simulink library "csu_cml_command_latch_lib"  (R2015b)
settings: Solver=ode45  StartTime=0.0  StopTime=10.0  RelTol=1e-3
values from neighbouring files (symbols this model uses):
  cml_mode_ids = zeros(size(cml_valid_modes))    [csu_cml_command_latch_init.m]
  cml_valid_mode_transitions = zeros(n, 'uint8')    [csu_cml_command_latch_init.m]
  csc_cmp_dt = fsw_dt    [csc_cmp_command_mode_process_init.m]
undefined symbols (not defined in the file or in its folder): cml_cmd_indices, cml_initial_value, cmp_msgid
libraries: simulink x8, util_event_lib x5, util_info_lib x1
settings Model: Creator=mstewart  LastModifiedBy=Mark Agbayani
settings DataIOCC: SaveFormat=Array
settings DebuggingCC: UnderspecifiedInitializationDetection=Classic  MergeDetectMultiDrivingBlocksExec=none  SolverPrmCheckMsg=warning  StateNameClashWarn=warning
settings HardwareCC: ProdBitPerPointer=32  ProdLargestAtomicFloat=None  ProdIntDivRoundTo=Undefined  ProdEndianess=Unspecified  ProdWordSize=32  ProdHWDeviceType=32-bit Generic
settings GRTTargetCC: GeneratePreprocessorConditionals=Disable all
settings ConfigComp: CovModelRefEnable=Off  CovSFcnEnable=off

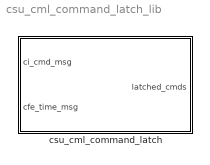
== system csu_cml_command_latch_lib ==
  csu_cml_command_latch : Subsystem

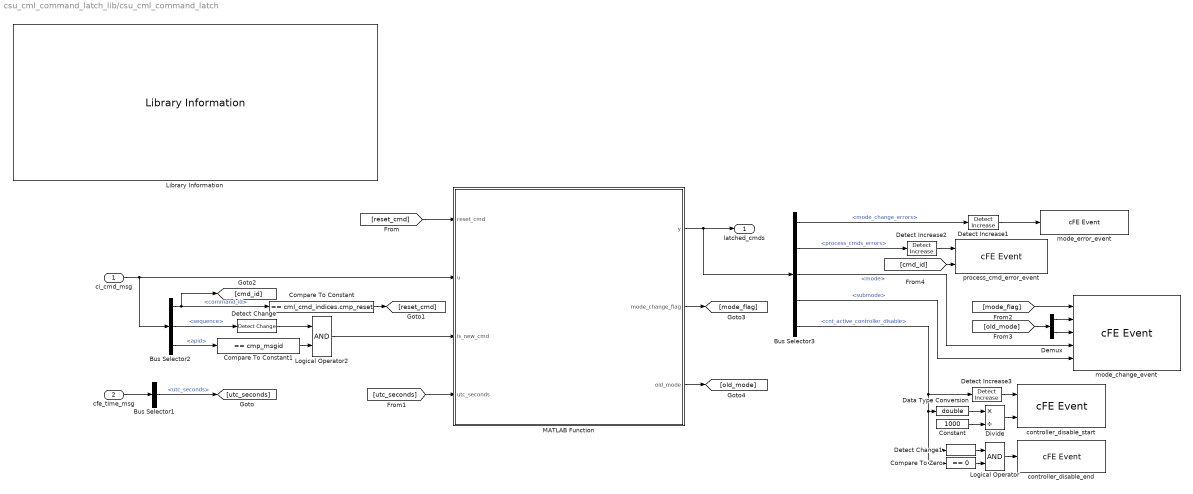
== system csu_cml_command_latch_lib/csu_cml_command_latch ==
  ci_cmd_msg : Inport  OutDataTypeStr=Bus: ci_cmd_msg
  cfe_time_msg : Inport  Port=2  OutDataTypeStr=Bus: cfe_time_msg
  Bus Selector1 : BusSelector  OutputSignals=utc_seconds
  Bus Selector2 : BusSelector  OutputSignals=command_id,sequence,apid
  Bus Selector3 : BusSelector  OutputSignals=mode_change_errors,process_cmds_errors,mode,submode,cnt_active_controller_disable
  Compare To Constant : simulink/Logic and Bit Operations/Compare To Constant  relop===  const=cml_cmd_indices.cmp_reset  OutDataTypeStr=boolean
  Compare To Constant1 : simulink/Logic and Bit Operations/Compare To Constant  relop===  const=cmp_msgid  OutDataTypeStr=boolean
  Compare To Zero : simulink/Logic and Bit Operations/Compare To Zero  relop===  OutDataTypeStr=boolean
  Constant : Constant  Value=1000  OutDataTypeStr=double
  Data Type Conversion : DataTypeConversion  OutDataTypeStr=double
  Demux : Demux  Outputs=2
  Detect Change : simulink/Logic and Bit Operations/Detect Change  vinit=0  InputProcessing=Inherited  OutDataTypeStr=boolean
  Detect Change1 : simulink/Logic and Bit Operations/Detect Change  vinit=0  InputProcessing=Inherited  OutDataTypeStr=boolean
  Detect Increase1 : simulink/Logic and Bit Operations/Detect Increase  vinit=0.0  InputProcessing=Inherited  OutDataTypeStr=boolean
  Detect Increase2 : simulink/Logic and Bit Operations/Detect Increase  vinit=0.0  InputProcessing=Inherited  OutDataTypeStr=boolean
  Detect Increase3 : simulink/Logic and Bit Operations/Detect Increase  vinit=0.0  InputProcessing=Inherited  OutDataTypeStr=boolean
  Divide : Product  Inputs=*/
  Library Information : util_info_lib/Library Information  owner='NONE'
  Logical Operator : Logic  AllPortsSameDT=off  OutDataTypeStr=boolean
  Logical Operator2 : Logic  AllPortsSameDT=off  OutDataTypeStr=boolean
  MATLAB Function : MATLAB Function  TreatAsAtomicUnit=on
  controller_disable_end : util_event_lib/cFE Event  event_message='Active Control Re-enabled'  event_id=24  event_severity=INFORMATION  event_filtered=off  event_mask=1  event_use_enums=off  event_enum_types={}
  controller_disable_start : util_event_lib/cFE Event  event_message='Active Control Disabled for %f seconds'  event_id=23  event_severity=INFORMATION  event_filtered=off  event_mask=1  event_use_enums=off  event_enum_types={}
  mode_change_event : util_event_lib/cFE Event  event_message='Mode changed from %s:%s to %s:%s'  event_id=20  event_severity=INFORMATION  event_filtered=off  event_mask=1  event_use_enums=on  event_enum_types={'enum_mode', 'enum_submode', 'enum_mode', 'enum_submode'}
  mode_error_event : util_event_lib/cFE Event  event_message='Invalid mode change requested'  event_id=22  event_severity=ERROR  event_filtered=off  event_mask=1  event_use_enums=off  event_enum_types={}
  process_cmd_error_event : util_event_lib/cFE Event  event_message='Error processing command with command code %u'  event_id=21  event_severity=ERROR  event_filtered=off  event_mask=1  event_use_enums=off  event_enum_types={}
  latched_cmds : Outport  OutDataTypeStr=Bus: cmp_bus_msg
  wires:
  Constant/1 -> Divide/2
  Data Type Conversion/1 -> Divide/1
  Divide/1 -> controller_disable_start/2
  Logical Operator/1 -> controller_disable_end/1
  Compare To Zero/1 -> Logical Operator/2
  Detect Change1/1 -> Logical Operator/1
  Bus Selector3/5 -> Detect Increase3/1, Compare To Zero/1, Detect Change1/1, Data Type Conversion/1  "<cnt_active_controller_disable>"
  Detect Increase3/1 -> controller_disable_start/1
  [old_mode] -> Demux/1
  [mode_flag] -> mode_change_event/1
  MATLAB Function/2(mode_change_flag) -> [mode_flag]
  Bus Selector3/4 -> mode_change_event/5  "<submode>"
  Bus Selector3/3 -> mode_change_event/4  "<mode>"
  Demux/2 -> mode_change_event/3
  Demux/1 -> mode_change_event/2
  ci_cmd_msg/1 -> MATLAB Function/2(u), Bus Selector2/1
  MATLAB Function/1(y) -> Bus Selector3/1, latched_cmds/1
  cfe_time_msg/1 -> Bus Selector1/1
  Bus Selector1/1 -> [utc_seconds]  "<utc_seconds>"
  Bus Selector2/1 -> [cmd_id], Compare To Constant/1  "<command_id>"
  Compare To Constant/1 -> [reset_cmd]
  Bus Selector2/2 -> Detect Change/1  "<sequence>"
  [reset_cmd] -> MATLAB Function/1(reset_cmd)
  [utc_seconds] -> MATLAB Function/4(utc_seconds)
  Logical Operator2/1 -> MATLAB Function/3(is_new_cmd)
  Bus Selector3/2 -> Detect Increase2/1  "<process_cmds_errors>"
  [cmd_id] -> process_cmd_error_event/2
  Detect Increase2/1 -> process_cmd_error_event/1
  Bus Selector3/1 -> Detect Increase1/1  "<mode_change_errors>"
  Detect Increase1/1 -> mode_error_event/1
  Bus Selector2/3 -> Compare To Constant1/1  "<apid>"
  Detect Change/1 -> Logical Operator2/1
  Compare To Constant1/1 -> Logical Operator2/2
  MATLAB Function/3(old_mode) -> [old_mode]

== matlab function csu_cml_command_latch_lib/csu_cml_command_latch/MATLAB Function ==
  data: csc_cmp_dt parameter; reset_cmd input boolean; u input Bus: ci_cmd_msg; y output Bus: cmp_bus_msg; is_new_cmd input boolean; utc_seconds input uint32; mode_change_flag output uint8; cml_valid_mode_transitions parameter; cml_mode_ids parameter uint8; cml_cmd_indices parameter; old_mode output uint8; cml_initial_value parameter
function [y, mode_change_flag, old_mode] = decode_and_latch(csc_cmp_dt, reset_cmd, u, is_new_cmd, utc_seconds, cml_valid_mode_transitions, cml_mode_ids, cml_cmd_indices, cml_initial_value)
%#codegen

persistent latched_values;
persistent internal_counters;

if isempty(latched_values)
    % load in inital values for all command signals
    latched_values = cml_initial_value;
end

if isempty(internal_counters)
    internal_counters.start_burn_count = uint8(0);
    internal_counters.old_mode = uint8( 1 );
    internal_counters.old_submode = uint8( 1 );
    internal_counters.controller_disable_counter = uint32( 0 );
    internal_counters.manual_thruster_duration_counter = uint32( zeros(26,1) );
    internal_counters.manual_thruster_arm_duration_counter = uint32( zeros(4,1) );
    internal_counters.act_reset = uint8(0);
end


if internal_counters.start_burn_count > 0
    internal_counters.start_burn_count = internal_counters.start_burn_count - 1;
    if internal_counters.start_burn_count == 0
        latched_values.start_burn = uint8(0);
    end
end

if internal_counters.act_reset > 0
    internal_counters.act_reset = internal_counters.act_reset - 1;
    if internal_counters.act_reset == 0
        latched_values.act_reset_accumulated_ontime = uint8(0);
    end
end

if internal_counters.controller_disable_counter > 0
    internal_counters.controller_disable_counter = internal_counters.controller_disable_counter - 100;
    if internal_counters.controller_disable_counter == 0
        latched_values.cnt_active_controller_disable = uint32(0);
    else
        latched_values.cnt_active_controller_disable = internal_counters.controller_disable_counter;
    end
end

if any(internal_counters.manual_thruster_duration_counter > 0)
    internal_counters.manual_thruster_duration_counter = max(internal_counters.manual_thruster_duration_counter - 100, uint32(zeros(26,1)));
    if all( internal_counters.manual_thruster_duration_counter == 0 )
        latched_values.act_manual_thruster_firing = uint32(zeros(26,1));
        internal_counters.manual_thruster_duration_counter = uint32(zeros(26,1));
    else
        latched_values.act_manual_thruster_firing = internal_counters.manual_thruster_duration_counter;
    end
end

if any(internal_counters.manual_thruster_arm_duration_counter > 0)
    internal_counters.manual_thruster_arm_duration_counter = max(internal_counters.manual_thruster_arm_duration_counter - 100, uint32(zeros(4,1)));
    if all( internal_counters.manual_thruster_arm_duration_counter == 0 )
        latched_values.act_arm_thruster_set_durations = uint32(zeros(4,1));
        internal_counters.manual_thruster_arm_duration_counter = uint32(zeros(4,1));
    else
        latched_values.act_arm_thruster_set_durations = internal_counters.manual_thruster_arm_duration_counter;
    end
end

old_mode = [ latched_values.mode latched_values.submode];
mode_change_flag = uint8( 0 );

if is_new_cmd
    
    latched_values.command_id = uint8(u.command_id);

    %%% Handle mode commands
    if (u.command_id == cml_cmd_indices.cmp_set_mode)

        new_mode = typecast(u.params(1),'uint8');   % decode requested "new mode"
        new_submode = typecast(u.params(2),'uint8');   % decode requested "new submode"
        
        if new_mode >= 1 && new_mode <= 9
            new_mode_id = cml_mode_ids(new_mode, new_submode);
            
            if new_mode_id ~= 0
                old_mode_id = cml_mode_ids(old_mode(1), old_mode(2));
                valid_mode_change = cml_valid_mode_transitions(old_mode_id, new_mode_id);
            else
                valid_mode_change = uint8(0);
            end
        else
            valid_mode_change = uint8(0);
        end

        if valid_mode_change                        % change modes

            latched_values.mode = new_mode;
            latched_values.submode = new_submode;
            
            if new_mode ~= internal_counters.old_mode || new_submode ~= internal_counters.old_submode
                mode_change_flag = uint8( 1 );
            end
            
            internal_counters.old_mode = new_mode;
            internal_counters.old_submode = new_submode;

            latched_values.mode_change_counter = latched_values.mode_change_counter + 1;

            if latched_values.cnt_active_controller_disable > 0     % If necessary, disable active_controller_disable
               latched_values.cnt_active_controller_disable = uint32(0);
               internal_counters.controller_disable_counter = uint32(0);
            end
            
            % If necessary, zero out current manual thruster commands
            if any(internal_counters.manual_thruster_duration_counter > 0)  || any(internal_counters.manual_thruster_arm_duration_counter > 0)
                latched_values.act_arm_thruster_set_durations = uint32(zeros(4,1));
                internal_counters.manual_thruster_arm_duration_counter = uint32(zeros(4,1));
                
                latched_values.act_manual_thruster_firing = uint32(zeros(26,1));
                internal_counters.manual_thruster_duration_counter = uint32(zeros(26,1));
            end

        else                                          % Invalid mode transition commanded, increment mode change errors counter

            latched_values.mode_change_errors = latched_values.mode_change_errors + 1;

        end                                           % Increment commands processed counter

        latched_values.process_cmds_counter = latched_values.process_cmds_counter + 1;

    elseif (u.command_id == cml_cmd_indices.cmp_disable_active_controller)
        latched_values.cnt_active_controller_disable = typecast(u.params(1:4),'uint32');
        internal_counters.controller_disable_counter = latched_values.cnt_active_controller_disable;
        
        % If necessary, zero out current manual thruster commands
        if any(internal_counters.manual_thruster_duration_counter > 0)  || any(internal_counters.manual_thruster_arm_duration_counter > 0)      
            latched_values.act_arm_thruster_set_durations = uint32(zeros(4,1));
            internal_counters.manual_thruster_arm_duration_counter = uint32(zeros(4,1));
            
            latched_values.act_manual_thruster_firing = uint32(zeros(26,1));
            internal_counters.manual_thruster_duration_counter = uint32(zeros(26,1));
        end
        
    elseif (u.command_id == cml_cmd_indices.cmp_reset_ctrs)
        latched_values.process_cmds_counter = uint16(0);
        latched_values.process_cmds_errors = uint16(0);
        latched_values.mode_change_counter = uint16(0);
        latched_values.mode_change_errors = uint16(0);
        
    elseif (u.command_id == cml_cmd_indices.gdn_hover_enable)
        latched_values.hover_enable = uint8(1);
        latched_values.process_cmds_counter = latched_values.process_cmds_counter + 1;
        
    elseif (u.command_id == cml_cmd_indices.gdn_hover_disable)
        latched_values.hover_enable = uint8(0);
        latched_values.process_cmds_counter = latched_values.process_cmds_counter + 1;
        
    elseif (u.command_id == cml_cmd_indices.gdn_takeoff_enable)
        latched_values.takeoff_enable = uint8(1);
        latched_values.process_cmds_counter = latched_values.process_cmds_counter + 1;
        
    elseif (u.command_id == cml_cmd_indices.gdn_takeoff_disable)
        latched_values.takeoff_enable = uint8(0);
        latched_values.process_cmds_counter = latched_values.process_cmds_counter + 1;
        
    elseif (u.command_id == cml_cmd_indices.gdn_set_burn_parameters)
        burn_type = typecast(u.params(1),'uint8');
        delta_v = typecast(u.params(2:9),'double');
        burn_dur = typecast(u.params(10:13),'single');
        
        if burn_type == 0 || burn_type == 1 || burn_type == 2 || burn_type == 3
            latched_values.burn_type_cmd = burn_type;
            latched_values.thruster_dv_cmd = delta_v;
            latched_values.thruster_dur_cmd = burn_dur;
        else
            latched_values.process_cmds_errors = latched_values.process_cmds_errors + 1;
        end
        
        latched_values.process_cmds_counter = latched_values.process_cmds_counter + 1;
        
    elseif (u.command_id == cml_cmd_indices.gdn_start_burn)
        
        if 1
            latched_values.start_burn = uint8(1);
            internal_counters.start_burn_count = uint8(1/csc_cmp_dt);
        else
            latched_values.process_cmds_errors = latched_values.process_cmds_errors + 1;
        end
        
        latched_values.process_cmds_counter = latched_values.process_cmds_counter + 1;
        
	elseif (u.command_id == cml_cmd_indices.gdn_set_inertial_primary_pointing_cmd)
        v_x = typecast(u.params(1:8),'double');
        v_y = typecast(u.params(9:16),'double');
        v_z = typecast(u.params(17:24),'double');
        
        if 1 % TODO: real error checking
            latched_values.inertial_primary_pointing_cmd = [v_x; v_y; v_z];
        else
            latched_values.process_cmds_errors = latched_values.process_cmds_errors + 1;
        end
        
        latched_values.process_cmds_counter = latched_values.process_cmds_counter + 1;
        
	elseif (u.command_id == cml_cmd_indices.gdn_set_inertial_secondary_pointing_cmd)
        v_x = typecast(u.params(1:8),'double');
        v_y = typecast(u.params(9:16),'double');
        v_z = typecast(u.params(17:24),'double');
        
        if 1 % TODO: real error checking
            latched_values.inertial_secondary_pointing_cmd = [v_x; v_y; v_z];
        else
            latched_values.process_cmds_errors = latched_values.process_cmds_errors + 1;
        end
        
        latched_values.process_cmds_counter = latched_values.process_cmds_counter + 1;
        
	elseif (u.command_id == cml_cmd_indices.gdn_set_body_secondary_pointing_vector)
        v_x = typecast(u.params(1:8),'double');
        v_y = typecast(u.params(9:16),'double');
        v_z = typecast(u.params(17:24),'double');
        
        if 1 % TODO: real error checking
            latched_values.body_secondary_pointing_vector = [v_x; v_y; v_z];
        else
            latched_values.process_cmds_errors = latched_values.process_cmds_errors + 1;
        end
        
        latched_values.process_cmds_counter = latched_values.process_cmds_counter + 1;
        
	elseif (u.command_id == cml_cmd_indices.gdn_set_body_primary_pointing_vector)
        v_x = typecast(u.params(1:8),'double');
        v_y = typecast(u.params(9:16),'double');
        v_z = typecast(u.params(17:24),'double');
        
        if 1 % TODO: real error checking
            latched_values.body_primary_pointing_vector = [v_x; v_y; v_z];
        else
            latched_values.process_cmds_errors = latched_values.process_cmds_errors + 1;
        end
        
        latched_values.process_cmds_counter = latched_values.process_cmds_counter + 1;
        
	elseif (u.command_id == cml_cmd_indices.gdn_set_peg_position_target)
        frame = typecast(u.params(1),'uint8');
        v_x = typecast(u.params(2:9),'double');
        v_y = typecast(u.params(10:17),'double');
        v_z = typecast(u.params(18:25),'double');
        
        if frame == 1 || frame == 3
            latched_values.peg_target_ref_frame = frame;
            latched_values.peg_position_target = [v_x; v_y; v_z];
        else
            latched_values.process_cmds_errors = latched_values.process_cmds_errors + 1;
        end
        
        latched_values.process_cmds_counter = latched_values.process_cmds_counter + 1;
                
	elseif (u.command_id == cml_cmd_indices.gdn_set_peg_velocity_target)
        frame = typecast(u.params(1),'uint8');
        v_x = typecast(u.params(2:9),'double');
        v_y = typecast(u.params(10:17),'double');
        v_z = typecast(u.params(18:25),'double');
        
        if frame == 1 || frame == 4
            latched_values.peg_target_ref_frame = frame;
            latched_values.peg_velocity_target = [v_x; v_y; v_z];
        else
            latched_values.process_cmds_errors = latched_values.process_cmds_errors + 1;
        end
        
        latched_values.process_cmds_counter = latched_values.process_cmds_counter + 1;
                
	elseif (u.command_id == cml_cmd_indices.gdn_set_vnc_primary_pointing_cmd)
        el = typecast(u.params(1:8),'double');
        az = typecast(u.params(9:16),'double');
        
        if 1 % TODO: real error checking
            latched_values.vnc_primary_pointing_cmd = [el; az];
        else
            latched_values.process_cmds_errors = latched_values.process_cmds_errors + 1;
        end
        
        latched_values.process_cmds_counter = latched_values.process_cmds_counter + 1;
        
    elseif (u.command_id == cml_cmd_indices.est_set_reference_frame)
        frame = typecast(u.params(1),'uint8');
        
        if 1 % TODO: real error checking
            latched_values.est_ref_frame = frame;
        else
            latched_values.process_cmds_errors = latched_values.process_cmds_errors + 1;
        end
        
        latched_values.process_cmds_counter = latched_values.process_cmds_counter + 1;
        
    elseif (u.command_id == cml_cmd_indices.cnt_select_thruster_set)
        thrusters = typecast(u.params(1),'uint8');
        
        if 1 % TODO: real error checking
            latched_values.acs_thruster_set = thrusters;
        else
            latched_values.process_cmds_errors = latched_values.process_cmds_errors + 1;
        end
        
        latched_values.process_cmds_counter = latched_values.process_cmds_counter + 1;
        
    
    elseif (u.command_id == cml_cmd_indices.act_fire_single_thruster)
        thruster_id = typecast(u.params(1),'uint8');
        duration = typecast(u.params(2:5),'uint32');
        
        if thruster_id > 0 && thruster_id <= 26 % TODO: real error checking

            latched_values.act_manual_thruster_firing(thruster_id) = uint32( duration );
                        
            internal_counters.manual_thruster_duration_counter = latched_values.act_manual_thruster_firing;
        else
            latched_values.act_manual_thruster_firing = uint32( zeros(26,1) );
        end
        
        latched_values.process_cmds_counter = latched_values.process_cmds_counter + 1;
        
    elseif (u.command_id == cml_cmd_indices.act_enable_thruster_set)

        thruster_set_id = typecast(u.params(1),'uint8');
        duration = typecast(u.params(2:5),'uint32');
        
        if thruster_set_id > 0 && thruster_set_id <= 4 % TODO: real error checking
            latched_values.act_arm_thruster_set_durations(thruster_set_id) = uint32( duration );
                        
            internal_counters.manual_thruster_arm_duration_counter = latched_values.act_arm_thruster_set_durations;
        else
            latched_values.act_arm_thruster_set_durations = uint32( zeros(4,1) );
        end
        
        latched_values.process_cmds_counter = latched_values.process_cmds_counter + 1;
        
    elseif (u.command_id == cml_cmd_indices.act_reset_accumulated_ontime)
        latched_values.act_reset_accumulated_ontime = uint8(1);
        latched_values.process_cmds_counter = latched_values.process_cmds_counter + 1;
        
        internal_counters.act_reset  = uint8(1);
        
   elseif (u.command_id == cml_cmd_indices.act_fire_coarse_thruster_pulse_zero_delay)
        coarse1  = typecast(u.params(1:4),'uint32');
        coarse2  = typecast(u.params(5:8),'uint32');
        coarse3  = typecast(u.params(9:12),'uint32');
        coarse4  = typecast(u.params(13:16),'uint32');
        coarse5  = typecast(u.params(17:20),'uint32');
        coarse6  = typecast(u.params(21:24),'uint32');
        coarse7  = typecast(u.params(25:28),'uint32');
        coarse8  = typecast(u.params(29:32),'uint32');
        coarse9  = typecast(u.params(33:36),'uint32');
        coarse10 = typecast(u.params(37:40),'uint32');
        coarse11 = typecast(u.params(41:44),'uint32');
        coarse12 = typecast(u.params(45:48),'uint32');

        if 1 % TODO: real error checking
            % cancels any previous manual commands when new is recevied
            latched_values.act_manual_thruster_firing(1)  = uint32( coarse1 );
            latched_values.act_manual_thruster_firing(2)  = uint32( coarse2 );
            latched_values.act_manual_thruster_firing(3)  = uint32( coarse3 );
            latched_values.act_manual_thruster_firing(4)  = uint32( coarse4 );
            latched_values.act_manual_thruster_firing(5)  = uint32( coarse5 );
            latched_values.act_manual_thruster_firing(6)  = uint32( coarse6 );
            latched_values.act_manual_thruster_firing(7)  = uint32( coarse7 );
            latched_values.act_manual_thruster_firing(8)  = uint32( coarse8 );
            latched_values.act_manual_thruster_firing(9)  = uint32( coarse9 );
            latched_values.act_manual_thruster_firing(10) = uint32( coarse10 );
            latched_values.act_manual_thruster_firing(11) = uint32( coarse11 );
            latched_values.act_manual_thruster_firing(12) = uint32( coarse12 );
                        
            internal_counters.manual_thruster_duration_counter = latched_values.act_manual_thruster_firing;
        else
            latched_values.act_manual_thruster_firing = uint32( zeros(26,1) );
        end
        
        latched_values.process_cmds_counter = latched_values.process_cmds_counter + 1;
    end
    
end

y = latched_values;
